simulink library "IOBlock_Library_TTC580"  (R2021a)
settings: Solver=ode45  StartTime=0.0  StopTime=10.0  RelTol=1e-3
PreLoadFcn:
  | addpath(genpath(fileparts(which('IOBlock_Library_TTC580'))));
  | %addpath(genpath(fileparts(which('IOBlock_Library_TTC580.mdl'))))
  | try
  | addpath(genpath([fileparts(which('IOBlock_Library_TTC580')),'\..\DBC_Importer']));
  | addpath(genpath([fileparts(which('IOBlock_Library_TTC580')),'\..\EEPROM_Importer']));
  | addpath(genpath([fileparts(which('IOBlock_Library_TTC580')),'\..\UserDoc']));
  | catch
  | warning('IOBlock_Library_TTC580: add path to DBC_Importer and EEPROM_Importer manually');
  | end
  | try
  | if exist('..\CustomPackage\scripts\OpenAllPackages.m','file')
  |      run('..\CustomPackage\scripts\OpenAllPackages.m'); %always available, ggf. empty
  | end
  | catch
  | warning('A problem occurred opening automatically the CustomPackage. Please open libraries manually');
  | end
  | try
  | set_param(0,'EditorSmartEditingHotParam','off');
  | catch
  | warning('Simlink preferences for ''Edit key parameter when adding new blocks'' needs to be unchecked manually');
  | end
undefined symbols (not defined in the file or in its folder): ADC_Absolute_10V, ADC_Absolute_32V, ADC_Absolute_5V, ADC_BoardTemp, ADC_ChannelInit, ADC_Current, ADC_Get, ADC_K15_, ADC_Ratiometric_10V, ADC_Ratiometric_5V, ADC_Resistive, ADC_SensorSupply, ADC_UBAT, bit_packing, bit_unpacking, CAN_ConfigMsg, compare2error, compare2FET_PROT_REENABLE, crc32_calc_intern, CRC32_EEPROM_Read, CRC32_EEPROM_Write, DIAG_EnterSafestate, DIAG_Status, DIAG_Status_internal, EEPROM_Mirror, EEPROM_Read, EEPROM_Read_OffsetIn, EEPROM_Read_Raw, EEPROM_Write, EEPROM_Write_OffsetIn, EEPROM_Write_Raw, EnterSafestate, FPU_Handler, Get_DI, Get_DI_VarThreshold, Get_K15_, Get_Pulse_Freq_Curr, Get_Pulse_Freq_Volt, Get_WakeUp, GetDateAndTime, IO_ADC_ResetProtection, IO_Blk_Lib_TTC500, IO_CAN_ReadMsg, IO_CAN_WriteMsg, IO_DI_Get, IO_DI_Init, IO_DI_Init_Var, IO_DO_GetCur, IO_DO_GetVoltage, IO_DO_Init, IO_DO_ResetProtection, IO_DO_Set, IO_Driver_GetSerialNumber, IO_Driver_GetVersionOfDriver, IO_Driver_GetVersionOfFPGA, IO_EEPROM_GetStatus, IO_EEPROM_Init, IO_EEPROM_Read_raw, IO_EEPROM_Write, IO_EEPROM_Write_OffsetIn ... (+73)
libraries: simulink x43
(part 1 of 18)
settings Model: ExtModeAutoUpdateStatusClock=off  Creator=hokka  LastModifiedBy=hokka
settings SolverCC: AlgebraicLoopSolver=TrustRegion
settings DataIOCC: LimitDataPoints=on  SaveFormat=Array  SignalLoggingSaveFormat=ModelDataLogs  ReturnWorkspaceOutputs=off
settings OptimizationCC: BlockReduction=off  BooleanDataType=off  LifeSpan=inf
settings DebuggingCC: SaveWithParameterizedLinksMsg=none  UnderspecifiedInitializationDetection=Classic  MergeDetectMultiDrivingBlocksExec=none  SignalResolutionControl=TryResolveAllWithWarning  SFUnexpectedBacktrackingDiag=warning  SFNoUnconditionalDefaultTransitionDiag=warning  SFExecutionAtInitializationDiag=none  SFMachineParentedDataDiag=warning  ArithmeticOperatorsInVariantConditions=warning
settings HardwareCC: ProdBitPerPointer=32  ProdBitPerSizeT=32  ProdBitPerPtrDiffT=32  ProdLargestAtomicFloat=None  ProdIntDivRoundTo=Undefined  ProdEndianess=Unspecified  ProdWordSize=32  ProdHWDeviceType=32-bit Generic  TargetUnknown=on
settings ModelReferenceCC: PropagateSignalLabelsOutOfModel=off
settings SFSimCC: SimUseLocalCustomCode=off  CustomCodeUndefinedFunction=UseInterfaceOnly
settings RTWCC: RTWUseLocalCustomCode=off
settings CodeAppCC: StateflowObjectComments=on
settings GRTTargetCC: TargetLangStandard=C89/C90 (ANSI)
settings ConfigComp: CovMetricSettings=dw  CovSaveCumulativeToWorkspaceVar=on  CovSaveSingleToWorkspaceVar=on  CovExternalEMLEnable=off  CovSFcnEnable=off

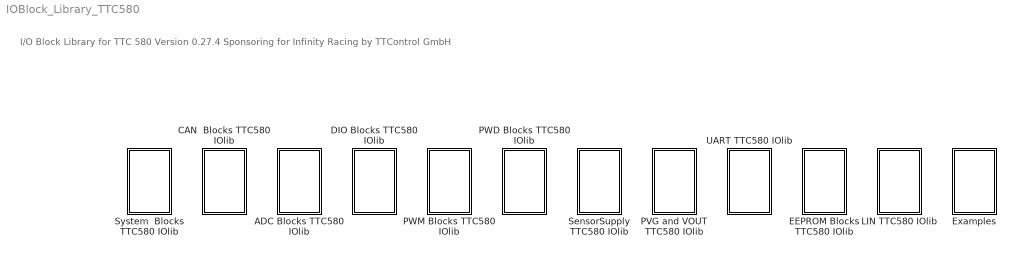
== system IOBlock_Library_TTC580 ==
  note: I/O Block Library for TTC 580
      | Version 0.27.4
      | Sponsoring for Infinity Racing by TTControl GmbH
  ADC Blocks TTC580 IOlib : Subsystem
  CAN  Blocks TTC580 IOlib : Subsystem
  DIO Blocks TTC580 IOlib : Subsystem
  EEPROM Blocks TTC580 IOlib : Subsystem
  Examples : Subsystem
  LIN TTC580 IOlib : Subsystem
  PVG and VOUT TTC580 IOlib : Subsystem
  PWD Blocks TTC580 IOlib : Subsystem
  PWM Blocks TTC580 IOlib : Subsystem
  SensorSupply TTC580 IOlib : Subsystem
  System  Blocks TTC580 IOlib : Subsystem
  UART TTC580 IOlib : Subsystem

== system IOBlock_Library_TTC580/ADC Blocks TTC580 IOlib ==
  ADC_Absolute_10V : Subsystem  LoadFcn=|  mask(ADC_Absolute_10V_Code){SampleTime=-1, ttlib=IO_Blk_Lib_TTC500, ttDescription=ADC_Absolute_10V, tt_iolib_version=0.26, adc_channel=IO_ADC_08, adc_type=IO_ADC_ABSOLUTE, range=IO_ADC_RANGE_10V, pupd=IO_ADC_NO_PULL, sensor_supply=IO_PIN_NONE}
      | try
      | %
      | %Upgrade Information - standard BEGIN
      | new_color = 'blue';
      | new_ver = '0.26';
      | act_ver = get_param(gcb,'tt_iolib_version');
      | if not(strcmp(act_ver,new_ver))
      |     disp(['Upgrade block: ',gcb,char(10),'       Version: ',act_ver,' to ',new_ver]);
      |     %switch - case for specific upgrade information e.g. additional parameter required 
      |     %Change appearance and version information
      |     set_param(gcb,'ForegroundColor',new_color);
      |     set_param(gcb,'tt_iolib_version',new_ver);
      | end
      | %Upgrade Information - standard END
      | catch
      | %Standard catch section BEGIN
      | errordlg('An error occurred in a callback of the TTC580-BlockLib. Please open the Diagnostic Viewer for further details');
      | disp(' ');
      | disp('------------------------------------------------------------');
      | disp('An error occurred in a callback of the TTC580-BlockLib.');
      | disp(['Please check the parameters in the mask of ',gcb]);
      | disp('If you do not encounter any violations, then please '); 
      | disp('copy the following lines and report this to support@ttcontrol.com ');
      | disp('<< begin of error message dump >>');
      | disp(['Version of TTC580-BlockLib: ', get_param(gcb,'tt_iolib_version')]);
      | disp(get_param(gcb,'ttDescription'));
      | disp(gcb);
      | x=lasterror;disp(x.message);
      | disp(get_param(gcb,'MaskValues'));
      | disp(version);
      | disp(computer);
      | disp('<< end of error message dump >>');
      | disp('------------------------------------------------------------');
      | disp(' ');
      | %Standard catch section END
      | end
      mask help: Returns the value of the given ADC channel: 0V..10V
      mask init:
      | try
      | %%CT>
      | TAG_loc = get_param(gcb,'Tag');
      | if ~isempty(TAG_loc),[~,y]=regexp(TAG_loc,'(^[a-zA-Z0-9_]*)');
      |     if isempty(y) || y~=builtin('length',(TAG_loc)) %don't use length() alone!
      |         error(['The Tag: ',TAG_loc,' needs to start with a letter and may only contain the characters 0-9,a-Z,_ .']);
      | end,end
      | x=find_system(gcbh,'FollowLinks','on','LookUnderMasks','on','BlockType','S-Function');
      | for i=1:builtin('length',(x)) %don't use length() alone!
      |     set_param(x(i),'Tag',TAG_loc);
      | end
      | %<CT%
      | 
      | catch
      | %Standard catch section BEGIN
      | errordlg('An error occurred in a callback of the TTC580-BlockLib. Please open the Diagnostic Viewer for further details');
      | disp(' ');
      | disp('------------------------------------------------------------');
      | disp('An error occurred in a callback of the TTC580-BlockLib.');
      | disp(['Please check the parameters in the mask of ',gcb]);
      | disp('If you do not encounter any violations, then please '); 
      | disp('copy the following lines and report this to support@ttcontrol.com ');
      | disp('<< begin of error message dump >>');
      | disp(['Version of TTC580-BlockLib: ', get_param(gcb,'tt_iolib_version')]);
      | disp(get_param(gcb,'ttDescription'));
      | disp(gcb);
      | x=lasterror;disp(x.message);
      | disp(get_param(gcb,'MaskValues'));
      | disp(version);
      | disp(computer);
      | disp('<< end of error message dump >>');
      | disp('------------------------------------------------------------');
      | disp(' ');
      | %Standard catch section END
      | end
      settings: CopyFcn=%deleted
      mask Help: web([which('usermanual.html'),'#',lower(get_param(gcb,'ttDescription'))])
      mask TypeOptions adc_channel: IO_ADC_08 | IO_ADC_09 | IO_ADC_10 | IO_ADC_11 | IO_ADC_12 | IO_ADC_13 | IO_ADC_14 | IO_ADC_15
      mask Callback adc_channel: %
      mask Callback adc_type: %
      mask Callback range: %
      mask Callback pupd: %
      mask Callback sensor_supply: %
  ADC_Absolute_32V : Subsystem  LoadFcn=|  mask(ADC_Absolute_32V_Code){SampleTime=-1, ttlib=IO_Blk_Lib_TTC500, ttDescription=ADC_Absolute_32V, tt_iolib_version=0.26, adc_channel=IO_ADC_16, adc_type=IO_ADC_ABSOLUTE, range=IO_ADC_RANGE_32V, pupd=IO_ADC_PD_10K, sensor_supply=IO_PIN_NONE}
      | try
      | %
      | %Upgrade Information - standard BEGIN
      | new_color = 'blue';
      | new_ver = '0.26';
      | act_ver = get_param(gcb,'tt_iolib_version');
      | if not(strcmp(act_ver,new_ver))
      |     disp(['Upgrade block: ',gcb,char(10),'       Version: ',act_ver,' to ',new_ver]);
      |     %switch - case for specific upgrade information e.g. additional parameter required 
      |     %Change appearance and version information
      |     set_param(gcb,'ForegroundColor',new_color);
      |     set_param(gcb,'tt_iolib_version',new_ver);
      | end
      | %Upgrade Information - standard END
      | catch
      | %Standard catch section BEGIN
      | errordlg('An error occurred in a callback of the TTC580-BlockLib. Please open the Diagnostic Viewer for further details');
      | disp(' ');
      | disp('------------------------------------------------------------');
      | disp('An error occurred in a callback of the TTC580-BlockLib.');
      | disp(['Please check the parameters in the mask of ',gcb]);
      | disp('If you do not encounter any violations, then please '); 
      | disp('copy the following lines and report this to support@ttcontrol.com ');
      | disp('<< begin of error message dump >>');
      | disp(['Version of TTC580-BlockLib: ', get_param(gcb,'tt_iolib_version')]);
      | disp(get_param(gcb,'ttDescription'));
      | disp(gcb);
      | x=lasterror;disp(x.message);
      | disp(get_param(gcb,'MaskValues'));
      | disp(version);
      | disp(computer);
      | disp('<< end of error message dump >>');
      | disp('------------------------------------------------------------');
      | disp(' ');
      | %Standard catch section END
      | end
      mask help: Returns the value of the given ADC channel: 0V..32V
      mask init: same as IOBlock_Library_TTC580/ADC Blocks TTC580 IOlib/ADC_Absolute_10V
      settings: CopyFcn=%deleted
      mask Help: web([which('usermanual.html'),'#',lower(get_param(gcb,'ttDescription'))])
      mask TypeOptions adc_channel: IO_ADC_16 | IO_ADC_17 | IO_ADC_18 | IO_ADC_19 | IO_ADC_20 | IO_ADC_21 | IO_ADC_22 | IO_ADC_23 | IO_ADC_24 | IO_ADC_25 | IO_ADC_26 | IO_ADC_27 | IO_ADC_28 | IO_ADC_29 | IO_ADC_30 | IO_ADC_31 | IO_ADC_32 | IO_ADC_33 | IO_ADC_34 | IO_ADC_35 | IO_ADC_36 | IO_ADC_37 | IO_ADC_38 | IO_ADC_39 | IO_ADC_40 | IO_ADC_41 | IO_ADC_42 | IO_ADC_43 | IO_ADC_44 | IO_ADC_45 | IO_ADC_46 | IO_ADC_47 | IO_ADC_48 | IO_ADC_49 | IO_ADC_50 | IO_ADC_51 | IO_ADC_52 | IO_ADC_53 | IO_ADC_54 | IO_ADC_55 | IO_ADC_56 | IO_ADC_57 | IO_ADC_58 | IO_ADC_59
      mask Callback adc_channel:
      | try
      | s_ParameterDecision = 'adc_channel'; %Deside on this parameter
      | cc_ValuesDecision={{'IO_ADC_16','IO_ADC_17','IO_ADC_18','IO_ADC_19','IO_ADC_20','IO_ADC_21','IO_ADC_22','IO_ADC_23'},{'IO_ADC_44','IO_ADC_45','IO_ADC_46','IO_ADC_47','IO_ADC_48','IO_ADC_49','IO_ADC_50','IO_ADC_51'}}; %Positive DescitionValues
      | s_ParameterGrey = 'pupd'; %Gray out this
      | c_ValueGrey = {'IO_ADC_PD_10K','IO_ADC_PU_10K'};   %Fixed value
      | %trim
      | s_ParameterDecision = strtrim(s_ParameterDecision);
      | cc_ValuesDecision = strtrim(cc_ValuesDecision);
      | s_ParameterGrey = strtrim(s_ParameterGrey);
      | c_ValueGrey = strtrim(c_ValueGrey);
      | c_MaskEnables=get_param(gcb,'MaskEnables');
      | %check consistency
      | if length(cc_ValuesDecision)~= length(c_ValueGrey),disp('DevCode: 012');end
      | idx=strmatch(s_ParameterGrey,get_param(gcb,'MaskNames'));
      | c_MaskEnables{idx}='on'; %default
      |     for i = 1: length(cc_ValuesDecision)
      |         if ~isempty(strmatch(get_param(gcb, s_ParameterDecision), cc_ValuesDecision{i},'exact'))
      |            set_param(gcb, s_ParameterGrey, c_ValueGrey{i});
      |            c_MaskEnables{idx}='off';
      |         end
      |     end
      | set_param(gcb,'MaskEnables',c_MaskEnables);
      | catch
      | %Standard catch section BEGIN
      | errordlg('An error occurred in a callback of the TTC580-BlockLib. Please open the Diagnostic Viewer for further details');
      | disp(' ');
      | disp('------------------------------------------------------------');
      | disp('An error occurred in a callback of the TTC580-BlockLib.');
      | disp(['Please check the parameters in the mask of ',gcb]);
      | disp('If you do not encounter any violations, then please ');
      | disp('copy the following lines and report this to support@ttcontrol.com ');
      | disp('<< begin of error message dump >>');
      | disp(['Version of TTC580-BlockLib: ', get_param(gcb,'tt_iolib_version')]);
      | disp(get_param(gcb,'ttDescription'));
      | disp(gcb);
      | x=lasterror;disp(x.message);
      | disp(get_param(gcb,'MaskValues'));
      | disp(version);
      | disp(computer);
      | disp('<< end of error message dump >>');
      | disp('------------------------------------------------------------');
      | disp(' ');
      | %Standard catch section END
      | end
      mask Callback adc_type: %
      mask Callback range: %
      mask TypeOptions pupd: IO_ADC_PU_10K | IO_ADC_PD_10K
      mask Callback pupd: %
      mask Callback sensor_supply: %
  ADC_Absolute_5V : Subsystem  LoadFcn=|  mask(ADC_Absolute_5V_Code){SampleTime=-1, ttlib=IO_Blk_Lib_TTC500, ttDescription=ADC_Absolute_5V, tt_iolib_version=0.26, adc_channel=IO_ADC_00, adc_type=IO_ADC_ABSOLUTE, range=IO_ADC_RANGE_5V, pupd=IO_ADC_NO_PULL, sensor_supply=IO_PIN_NONE}
      | try
      | %
      | %Upgrade Information - standard BEGIN
      | new_color = 'blue';
      | new_ver = '0.26';
      | act_ver = get_param(gcb,'tt_iolib_version');
      | if not(strcmp(act_ver,new_ver))
      |     disp(['Upgrade block: ',gcb,char(10),'       Version: ',act_ver,' to ',new_ver]);
      |     %switch - case for specific upgrade information e.g. additional parameter required 
      |     %Change appearance and version information
      |     set_param(gcb,'ForegroundColor',new_color);
      |     set_param(gcb,'tt_iolib_version',new_ver);
      | end
      | %Upgrade Information - standard END
      | catch
      | %Standard catch section BEGIN
      | errordlg('An error occurred in a callback of the TTC580-BlockLib. Please open the Diagnostic Viewer for further details');
      | disp(' ');
      | disp('------------------------------------------------------------');
      | disp('An error occurred in a callback of the TTC580-BlockLib.');
      | disp(['Please check the parameters in the mask of ',gcb]);
      | disp('If you do not encounter any violations, then please '); 
      | disp('copy the following lines and report this to support@ttcontrol.com ');
      | disp('<< begin of error message dump >>');
      | disp(['Version of TTC580-BlockLib: ', get_param(gcb,'tt_iolib_version')]);
      | disp(get_param(gcb,'ttDescription'));
      | disp(gcb);
      | x=lasterror;disp(x.message);
      | disp(get_param(gcb,'MaskValues'));
      | disp(version);
      | disp(computer);
      | disp('<< end of error message dump >>');
      | disp('------------------------------------------------------------');
      | disp(' ');
      | %Standard catch section END
      | end
      mask help: Returns the value of the given ADC channel: 0V..5V
      mask init: same as IOBlock_Library_TTC580/ADC Blocks TTC580 IOlib/ADC_Absolute_10V
      settings: CopyFcn=%deleted
      mask Help: web([which('usermanual.html'),'#',lower(get_param(gcb,'ttDescription'))])
      mask TypeOptions adc_channel: IO_ADC_00 | IO_ADC_01 | IO_ADC_02 | IO_ADC_03 | IO_ADC_04 | IO_ADC_05 | IO_ADC_06 | IO_ADC_07 | IO_ADC_08 | IO_ADC_09 | IO_ADC_10 | IO_ADC_11 | IO_ADC_12 | IO_ADC_13 | IO_ADC_14 | IO_ADC_15 | IO_ADC_16 | IO_ADC_17 | IO_ADC_18 | IO_ADC_19 | IO_ADC_20 | IO_ADC_21 | IO_ADC_22 | IO_ADC_23
      mask Callback adc_channel: %
      mask Callback adc_type: %
      mask Callback range: %
      mask Callback pupd: %
      mask Callback sensor_supply: %
  ADC_BoardTemp : Subsystem  LoadFcn=|  mask(ADC_BoardTemp_Code){SampleTime=-1, ttlib=IO_Blk_Lib_TTC500, ttDescription=ADC_BoardTemp, tt_iolib_version=0.26, adc_channel=IO_ADC_BOARD_TEMP, adc_type=IO_ADC_ABSOLUTE, range=IO_ADC_RANGE_32V, pupd=IO_ADC_NO_PULL, sensor_supply=IO_PIN_NONE}
      | try
      | %
      | %Upgrade Information - standard BEGIN
      | new_color = 'blue';
      | new_ver = '0.26';
      | act_ver = get_param(gcb,'tt_iolib_version');
      | if not(strcmp(act_ver,new_ver))
      |     disp(['Upgrade block: ',gcb,char(10),'       Version: ',act_ver,' to ',new_ver]);
      |     %switch - case for specific upgrade information e.g. additional parameter required 
      |     %Change appearance and version information
      |     set_param(gcb,'ForegroundColor',new_color);
      |     set_param(gcb,'tt_iolib_version',new_ver);
      | end
      | %Upgrade Information - standard END
      | catch
      | %Standard catch section BEGIN
      | errordlg('An error occurred in a callback of the TTC580-BlockLib. Please open the Diagnostic Viewer for further details');
      | disp(' ');
      | disp('------------------------------------------------------------');
      | disp('An error occurred in a callback of the TTC580-BlockLib.');
      | disp(['Please check the parameters in the mask of ',gcb]);
      | disp('If you do not encounter any violations, then please '); 
      | disp('copy the following lines and report this to support@ttcontrol.com ');
      | disp('<< begin of error message dump >>');
      | disp(['Version of TTC580-BlockLib: ', get_param(gcb,'tt_iolib_version')]);
      | disp(get_param(gcb,'ttDescription'));
      | disp(gcb);
      | x=lasterror;disp(x.message);
      | disp(get_param(gcb,'MaskValues'));
      | disp(version);
      | disp(computer);
      | disp('<< end of error message dump >>');
      | disp('------------------------------------------------------------');
      | disp(' ');
      | %Standard catch section END
      | end
      mask help: Returns the value of the board temperature: -63°C .. 152°C
      mask init: same as IOBlock_Library_TTC580/ADC Blocks TTC580 IOlib/ADC_Absolute_10V
      settings: CopyFcn=%deleted
      mask Help: web([which('usermanual.html'),'#',lower(get_param(gcb,'ttDescription'))])
      mask Callback adc_channel: %
      mask Callback adc_type: %
      mask Callback range: %
      mask Callback pupd: %
      mask Callback sensor_supply: %
  ADC_Current : Subsystem  LoadFcn=|  mask(ADC_Current_Code){SampleTime=-1, ttlib=IO_Blk_Lib_TTC500, ttDescription=ADC_Current, tt_iolib_version=0.26, adc_channel=IO_ADC_00, adc_type=IO_ADC_CURRENT, range=IO_ADC_NO_RANGE, pupd=IO_ADC_NO_PULL, sensor_supply=IO_PIN_NONE}
      | try
      | %
      | %Upgrade Information - standard BEGIN
      | new_color = 'blue';
      | new_ver = '0.26';
      | act_ver = get_param(gcb,'tt_iolib_version');
      | if not(strcmp(act_ver,new_ver))
      |     disp(['Upgrade block: ',gcb,char(10),'       Version: ',act_ver,' to ',new_ver]);
      |     %switch - case for specific upgrade information e.g. additional parameter required 
      |     %Change appearance and version information
      |     set_param(gcb,'ForegroundColor',new_color);
      |     set_param(gcb,'tt_iolib_version',new_ver);
      | end
      | %Upgrade Information - standard END
      | catch
      | %Standard catch section BEGIN
      | errordlg('An error occurred in a callback of the TTC580-BlockLib. Please open the Diagnostic Viewer for further details');
      | disp(' ');
      | disp('------------------------------------------------------------');
      | disp('An error occurred in a callback of the TTC580-BlockLib.');
      | disp(['Please check the parameters in the mask of ',gcb]);
      | disp('If you do not encounter any violations, then please '); 
      | disp('copy the following lines and report this to support@ttcontrol.com ');
      | disp('<< begin of error message dump >>');
      | disp(['Version of TTC580-BlockLib: ', get_param(gcb,'tt_iolib_version')]);
      | disp(get_param(gcb,'ttDescription'));
      | disp(gcb);
      | x=lasterror;disp(x.message);
      | disp(get_param(gcb,'MaskValues'));
      | disp(version);
      | disp(computer);
      | disp('<< end of error message dump >>');
      | disp('------------------------------------------------------------');
      | disp(' ');
      | %Standard catch section END
      | end
      mask help: Returns the value of the given ADC channel: 0mA..25mA
      mask init: same as IOBlock_Library_TTC580/ADC Blocks TTC580 IOlib/ADC_Absolute_10V
      settings: CopyFcn=%deleted
      mask Help: web([which('usermanual.html'),'#',lower(get_param(gcb,'ttDescription'))])
      mask TypeOptions adc_channel: IO_ADC_00 | IO_ADC_01 | IO_ADC_02 | IO_ADC_03 | IO_ADC_04 | IO_ADC_05 | IO_ADC_06 | IO_ADC_07 | IO_ADC_08 | IO_ADC_09 | IO_ADC_10 | IO_ADC_11 | IO_ADC_12 | IO_ADC_13 | IO_ADC_14 | IO_ADC_15 | IO_ADC_16 | IO_ADC_17 | IO_ADC_18 | IO_ADC_19 | IO_ADC_20 | IO_ADC_21 | IO_ADC_22 | IO_ADC_23
      mask Callback adc_channel: %
      mask Callback adc_type: %
      mask Callback range: %
      mask Callback pupd: %
      mask Callback sensor_supply: %
  ADC_K15_ : Subsystem  LoadFcn=|  mask(ADC_K15__Code){SampleTime=-1, ttlib=IO_Blk_Lib_TTC500, ttDescription=ADC_K15_, tt_iolib_version=0.26, adc_channel=IO_ADC_K15, adc_type=IO_ADC_ABSOLUTE, range=IO_ADC_RANGE_32V, pupd=IO_ADC_NO_PULL, sensor_supply=IO_PIN_NONE}
      | try
      | %
      | %Upgrade Information - standard BEGIN
      | new_color = 'blue';
      | new_ver = '0.26';
      | act_ver = get_param(gcb,'tt_iolib_version');
      | if not(strcmp(act_ver,new_ver))
      |     disp(['Upgrade block: ',gcb,char(10),'       Version: ',act_ver,' to ',new_ver]);
      |     %switch - case for specific upgrade information e.g. additional parameter required 
      |     %Change appearance and version information
      |     set_param(gcb,'ForegroundColor',new_color);
      |     set_param(gcb,'tt_iolib_version',new_ver);
      | end
      | %Upgrade Information - standard END
      | catch
      | %Standard catch section BEGIN
      | errordlg('An error occurred in a callback of the TTC580-BlockLib. Please open the Diagnostic Viewer for further details');
      | disp(' ');
      | disp('------------------------------------------------------------');
      | disp('An error occurred in a callback of the TTC580-BlockLib.');
      | disp(['Please check the parameters in the mask of ',gcb]);
      | disp('If you do not encounter any violations, then please '); 
      | disp('copy the following lines and report this to support@ttcontrol.com ');
      | disp('<< begin of error message dump >>');
      | disp(['Version of TTC580-BlockLib: ', get_param(gcb,'tt_iolib_version')]);
      | disp(get_param(gcb,'ttDescription'));
      | disp(gcb);
      | x=lasterror;disp(x.message);
      | disp(get_param(gcb,'MaskValues'));
      | disp(version);
      | disp(computer);
      | disp('<< end of error message dump >>');
      | disp('------------------------------------------------------------');
      | disp(' ');
      | %Standard catch section END
      | end
      mask help: Returns the value of the Terminal 15 Input channel: 0V..55V
      mask init: same as IOBlock_Library_TTC580/ADC Blocks TTC580 IOlib/ADC_Absolute_10V
      settings: CopyFcn=%deleted
      mask Help: web([which('usermanual.html'),'#',lower(get_param(gcb,'ttDescription'))])
      mask Callback adc_channel: %
      mask Callback adc_type: %
      mask Callback range: %
      mask Callback pupd: %
      mask Callback sensor_supply: %
  ADC_Ratiometric_10V : Subsystem  LoadFcn=|  mask(ADC_Ratiometric_10V_Code){SampleTime=-1, ttlib=IO_Blk_Lib_TTC500, ttDescription=ADC_Ratiometric_10V, tt_iolib_version=0.26, adc_channel=IO_ADC_08, adc_type=IO_ADC_RATIOMETRIC, range=IO_ADC_RANGE_10V, pupd=IO_ADC_NO_PULL, sensor_supply=IO_SENSOR_SUPPLY_2, volt_sensor_supply=IO_POWER_ON_5V}
      | try
      | %
      | %Upgrade Information - standard BEGIN
      | new_color = 'blue';
      | new_ver = '0.26';
      | act_ver = get_param(gcb,'tt_iolib_version');
      | if not(strcmp(act_ver,new_ver))
      |     disp(['Upgrade block: ',gcb,char(10),'       Version: ',act_ver,' to ',new_ver]);
      |     %switch - case for specific upgrade information e.g. additional parameter required 
      |     %Change appearance and version information
      |     set_param(gcb,'ForegroundColor',new_color);
      |     set_param(gcb,'tt_iolib_version',new_ver);
      | end
      | %Upgrade Information - standard END
      | catch
      | %Standard catch section BEGIN
      | errordlg('An error occurred in a callback of the TTC580-BlockLib. Please open the Diagnostic Viewer for further details');
      | disp(' ');
      | disp('------------------------------------------------------------');
      | disp('An error occurred in a callback of the TTC580-BlockLib.');
      | disp(['Please check the parameters in the mask of ',gcb]);
      | disp('If you do not encounter any violations, then please '); 
      | disp('copy the following lines and report this to support@ttcontrol.com ');
      | disp('<< begin of error message dump >>');
      | disp(['Version of TTC580-BlockLib: ', get_param(gcb,'tt_iolib_version')]);
      | disp(get_param(gcb,'ttDescription'));
      | disp(gcb);
      | x=lasterror;disp(x.message);
      | disp(get_param(gcb,'MaskValues'));
      | disp(version);
      | disp(computer);
      | disp('<< end of error message dump >>');
      | disp('------------------------------------------------------------');
      | disp(' ');
      | %Standard catch section END
      | end
      mask help: Returns the value of the given ADC channel: 0V..10V
      mask init: same as IOBlock_Library_TTC580/ADC Blocks TTC580 IOlib/ADC_Absolute_10V
      settings: CopyFcn=%deleted
      mask Help: web([which('usermanual.html'),'#',lower(get_param(gcb,'ttDescription'))])
      mask TypeOptions adc_channel: IO_ADC_08 | IO_ADC_09 | IO_ADC_10 | IO_ADC_11 | IO_ADC_12 | IO_ADC_13 | IO_ADC_14 | IO_ADC_15
      mask Callback adc_channel: %
      mask Callback adc_type: %
      mask Callback range: %
      mask Callback pupd: %
      mask Callback sensor_supply: %
      mask TypeOptions volt_sensor_supply: IO_POWER_ON_5V | IO_POWER_ON_6V | IO_POWER_ON_7V | IO_POWER_ON_8V | IO_POWER_ON_9V | IO_POWER_ON_10V
      mask Callback volt_sensor_supply: %
  ADC_Ratiometric_5V : Subsystem  LoadFcn=|  mask(ADC_Ratiometric_5V_Code){SampleTime=-1, ttlib=IO_Blk_Lib_TTC500, ttDescription=ADC_Ratiometric_5V, tt_iolib_version=0.25, adc_channel=IO_ADC_00, adc_type=IO_ADC_RATIOMETRIC, range=IO_ADC_RANGE_5V, pupd=IO_ADC_NO_PULL, sensor_supply=IO_SENSOR_SUPPLY_0}
      | try
      | %
      | %Upgrade Information - standard BEGIN
      | new_color = 'blue';
      | new_ver = '0.25';
      | act_ver = get_param(gcb,'tt_iolib_version');
      | if not(strcmp(act_ver,new_ver))
      |     disp(['Upgrade block: ',gcb,char(10),'       Version: ',act_ver,' to ',new_ver]);
      |     %switch - case for specific upgrade information e.g. additional parameter required 
      |     %Change appearance and version information
      |     set_param(gcb,'ForegroundColor',new_color);
      |     set_param(gcb,'tt_iolib_version',new_ver);
      | end
      | %Upgrade Information - standard END
      | catch
      | %Standard catch section BEGIN
      | errordlg('An error occurred in a callback of the TTC580-BlockLib. Please open the Diagnostic Viewer for further details');
      | disp(' ');
      | disp('------------------------------------------------------------');
      | disp('An error occurred in a callback of the TTC580-BlockLib.');
      | disp(['Please check the parameters in the mask of ',gcb]);
      | disp('If you do not encounter any violations, then please '); 
      | disp('copy the following lines and report this to support@ttcontrol.com ');
      | disp('<< begin of error message dump >>');
      | disp(['Version of TTC580-BlockLib: ', get_param(gcb,'tt_iolib_version')]);
      | disp(get_param(gcb,'ttDescription'));
      | disp(gcb);
      | x=lasterror;disp(x.message);
      | disp(get_param(gcb,'MaskValues'));
      | disp(version);
      | disp(computer);
      | disp('<< end of error message dump >>');
      | disp('------------------------------------------------------------');
      | disp(' ');
      | %Standard catch section END
      | end
      mask help: Returns the value of the given ADC channel: 0V..5V
      mask init:
      | try
      | switch sensor_supply
      |    case {'IO_SENSOR_SUPPLY_0','IO_SENSOR_SUPPLY_1'}
      |       volt_sensor_supply = 'IO_POWER_ON';
      |    case {'IO_SENSOR_SUPPLY_2'}
      |       volt_sensor_supply = 'IO_POWER_ON_5V';
      |    otherwise
      |       error('Wrong option for sensor_supply');
      | end
      | %%CT>
      | TAG_loc = get_param(gcb,'Tag');
      | if ~isempty(TAG_loc),[~,y]=regexp(TAG_loc,'(^[a-zA-Z0-9_]*)');
      |     if isempty(y) || y~=builtin('length',(TAG_loc)) %don't use length() alone!
      |         error(['The Tag: ',TAG_loc,' needs to start with a letter and may only contain the characters 0-9,a-Z,_ .']);
      | end,end
      | x=find_system(gcbh,'FollowLinks','on','LookUnderMasks','on','BlockType','S-Function');
      | for i=1:builtin('length',(x)) %don't use length() alone!
      |     set_param(x(i),'Tag',TAG_loc);
      | end
      | %<CT%
      | 
      | catch
      | %Standard catch section BEGIN
      | errordlg('An error occurred in a callback of the TTC580-BlockLib. Please open the Diagnostic Viewer for further details');
      | disp(' ');
      | disp('------------------------------------------------------------');
      | disp('An error occurred in a callback of the TTC580-BlockLib.');
      | disp(['Please check the parameters in the mask of ',gcb]);
      | disp('If you do not encounter any violations, then please '); 
      | disp('copy the following lines and report this to support@ttcontrol.com ');
      | disp('<< begin of error message dump >>');
      | disp(['Version of TTC580-BlockLib: ', get_param(gcb,'tt_iolib_version')]);
      | disp(get_param(gcb,'ttDescription'));
      | disp(gcb);
      | x=lasterror;disp(x.message);
      | disp(get_param(gcb,'MaskValues'));
      | disp(version);
      | disp(computer);
      | disp('<< end of error message dump >>');
      | disp('------------------------------------------------------------');
      | disp(' ');
      | %Standard catch section END
      | end
      settings: CopyFcn=%deleted
      mask Help: web([which('usermanual.html'),'#',lower(get_param(gcb,'ttDescription'))])
      mask TypeOptions adc_channel: IO_ADC_00 | IO_ADC_01 | IO_ADC_02 | IO_ADC_03 | IO_ADC_04 | IO_ADC_05 | IO_ADC_06 | IO_ADC_07 | IO_ADC_08 | IO_ADC_09 | IO_ADC_10 | IO_ADC_11 | IO_ADC_12 | IO_ADC_13 | IO_ADC_14 | IO_ADC_15 | IO_ADC_16 | IO_ADC_17 | IO_ADC_18 | IO_ADC_19 | IO_ADC_20 | IO_ADC_21 | IO_ADC_22 | IO_ADC_23
      mask Callback adc_channel: %
      mask Callback adc_type: %
      mask Callback range: %
      mask Callback pupd: %
      mask TypeOptions sensor_supply: IO_SENSOR_SUPPLY_0 | IO_SENSOR_SUPPLY_1 | IO_SENSOR_SUPPLY_2
      mask Callback sensor_supply: %
  ADC_Resistive : Subsystem  LoadFcn=|  mask(ADC_Resistive_Code){SampleTime=-1, ttlib=IO_Blk_Lib_TTC500, ttDescription=ADC_Resistive, tt_iolib_version=0.26, adc_channel=IO_ADC_00, adc_type=IO_ADC_RESISTIVE, range=IO_ADC_NO_RANGE, pupd=IO_ADC_NO_PULL, sensor_supply=IO_PIN_NONE}
      | try
      | %
      | %Upgrade Information - standard BEGIN
      | new_color = 'blue';
      | new_ver = '0.26';
      | act_ver = get_param(gcb,'tt_iolib_version');
      | if not(strcmp(act_ver,new_ver))
      |     disp(['Upgrade block: ',gcb,char(10),'       Version: ',act_ver,' to ',new_ver]);
      |     %switch - case for specific upgrade information e.g. additional parameter required 
      |     %Change appearance and version information
      |     set_param(gcb,'ForegroundColor',new_color);
      |     set_param(gcb,'tt_iolib_version',new_ver);
      | end
      | %Upgrade Information - standard END
      | catch
      | %Standard catch section BEGIN
      | errordlg('An error occurred in a callback of the TTC580-BlockLib. Please open the Diagnostic Viewer for further details');
      | disp(' ');
      | disp('------------------------------------------------------------');
      | disp('An error occurred in a callback of the TTC580-BlockLib.');
      | disp(['Please check the parameters in the mask of ',gcb]);
      | disp('If you do not encounter any violations, then please '); 
      | disp('copy the following lines and report this to support@ttcontrol.com ');
      | disp('<< begin of error message dump >>');
      | disp(['Version of TTC580-BlockLib: ', get_param(gcb,'tt_iolib_version')]);
      | disp(get_param(gcb,'ttDescription'));
      | disp(gcb);
      | x=lasterror;disp(x.message);
      | disp(get_param(gcb,'MaskValues'));
      | disp(version);
      | disp(computer);
      | disp('<< end of error message dump >>');
      | disp('------------------------------------------------------------');
      | disp(' ');
      | %Standard catch section END
      | end
      mask help: Returns the value of the given ADC channel: 0Ohm..100000Ohm
      mask init: same as IOBlock_Library_TTC580/ADC Blocks TTC580 IOlib/ADC_Absolute_10V
      settings: CopyFcn=%deleted
      mask Help: web([which('usermanual.html'),'#',lower(get_param(gcb,'ttDescription'))])
      mask TypeOptions adc_channel: IO_ADC_00 | IO_ADC_01 | IO_ADC_02 | IO_ADC_03 | IO_ADC_04 | IO_ADC_05 | IO_ADC_06 | IO_ADC_07
      mask Callback adc_channel: %
      mask Callback adc_type: %
      mask Callback range: %
      mask Callback pupd: %
      mask Callback sensor_supply: %
  ADC_SensorSupply : Subsystem  LoadFcn=|  mask(ADC_SensorSupply_Code){SampleTime=-1, ttlib=IO_Blk_Lib_TTC500, ttDescription=ADC_SensorSupply, tt_iolib_version=0.26, adc_channel=IO_ADC_SENSOR_SUPPLY_0, adc_type=IO_ADC_ABSOLUTE, range=IO_ADC_RANGE_32V, pupd=IO_ADC_NO_PULL, sensor_supply=IO_PIN_NONE}
      | try
      | %
      | %Upgrade Information - standard BEGIN
      | new_color = 'blue';
      | new_ver = '0.26';
      | act_ver = get_param(gcb,'tt_iolib_version');
      | if not(strcmp(act_ver,new_ver))
      |     disp(['Upgrade block: ',gcb,char(10),'       Version: ',act_ver,' to ',new_ver]);
      |     %switch - case for specific upgrade information e.g. additional parameter required 
      |     %Change appearance and version information
      |     set_param(gcb,'ForegroundColor',new_color);
      |     set_param(gcb,'tt_iolib_version',new_ver);
      | end
      | %Upgrade Information - standard END
      | catch
      | %Standard catch section BEGIN
      | errordlg('An error occurred in a callback of the TTC580-BlockLib. Please open the Diagnostic Viewer for further details');
      | disp(' ');
      | disp('------------------------------------------------------------');
      | disp('An error occurred in a callback of the TTC580-BlockLib.');
      | disp(['Please check the parameters in the mask of ',gcb]);
      | disp('If you do not encounter any violations, then please '); 
      | disp('copy the following lines and report this to support@ttcontrol.com ');
      | disp('<< begin of error message dump >>');
      | disp(['Version of TTC580-BlockLib: ', get_param(gcb,'tt_iolib_version')]);
      | disp(get_param(gcb,'ttDescription'));
      | disp(gcb);
      | x=lasterror;disp(x.message);
      | disp(get_param(gcb,'MaskValues'));
      | disp(version);
      | disp(computer);
      | disp('<< end of error message dump >>');
      | disp('------------------------------------------------------------');
      | disp(' ');
      | %Standard catch section END
      | end
      mask help: Returns the value of the associated sensor supply ADC channel: 0V..10.560V
      mask init: same as IOBlock_Library_TTC580/ADC Blocks TTC580 IOlib/ADC_Absolute_10V
      settings: CopyFcn=%deleted
      mask Help: web([which('usermanual.html'),'#',lower(get_param(gcb,'ttDescription'))])
      mask TypeOptions adc_channel: IO_ADC_SENSOR_SUPPLY_0 | IO_ADC_SENSOR_SUPPLY_1 | IO_ADC_SENSOR_SUPPLY_2
      mask Callback adc_channel: %
      mask Callback adc_type: %
      mask Callback range: %
      mask Callback pupd: %
      mask Callback sensor_supply: %
  ADC_UBAT : Subsystem  LoadFcn=|  mask(ADC_UBAT_Code){SampleTime=-1, ttlib=IO_Blk_Lib_TTC500, ttDescription=ADC_UBAT, tt_iolib_version=0.26, adc_channel=IO_ADC_UBAT, adc_type=IO_ADC_ABSOLUTE, range=IO_ADC_RANGE_32V, pupd=IO_ADC_NO_PULL, sensor_supply=IO_PIN_NONE}
      | try
      | %
      | %Upgrade Information - standard BEGIN
      | new_color = 'blue';
      | new_ver = '0.26';
      | act_ver = get_param(gcb,'tt_iolib_version');
      | if not(strcmp(act_ver,new_ver))
      |     disp(['Upgrade block: ',gcb,char(10),'       Version: ',act_ver,' to ',new_ver]);
      |     %switch - case for specific upgrade information e.g. additional parameter required 
      |     %Change appearance and version information
      |     set_param(gcb,'ForegroundColor',new_color);
      |     set_param(gcb,'tt_iolib_version',new_ver);
      | end
      | %Upgrade Information - standard END
      | catch
      | %Standard catch section BEGIN
      | errordlg('An error occurred in a callback of the TTC580-BlockLib. Please open the Diagnostic Viewer for further details');
      | disp(' ');
      | disp('------------------------------------------------------------');
      | disp('An error occurred in a callback of the TTC580-BlockLib.');
      | disp(['Please check the parameters in the mask of ',gcb]);
      | disp('If you do not encounter any violations, then please '); 
      | disp('copy the following lines and report this to support@ttcontrol.com ');
      | disp('<< begin of error message dump >>');
      | disp(['Version of TTC580-BlockLib: ', get_param(gcb,'tt_iolib_version')]);
      | disp(get_param(gcb,'ttDescription'));
      | disp(gcb);
      | x=lasterror;disp(x.message);
      | disp(get_param(gcb,'MaskValues'));
      | disp(version);
      | disp(computer);
      | disp('<< end of error message dump >>');
      | disp('------------------------------------------------------------');
      | disp(' ');
      | %Standard catch section END
      | end
      mask help: Returns the value of the battery ADC channel: 0V..55V
      mask init: same as IOBlock_Library_TTC580/ADC Blocks TTC580 IOlib/ADC_Absolute_10V
      settings: CopyFcn=%deleted
      mask Help: web([which('usermanual.html'),'#',lower(get_param(gcb,'ttDescription'))])
      mask Callback adc_channel: %
      mask Callback adc_type: %
      mask Callback range: %
      mask Callback pupd: %
      mask Callback sensor_supply: %
